simulink model "PID_Board"  (R2020b)
settings: Solver=ode3  StartTime=0.0  StopTime=inf  FixedStep=0.001  RelTol=1e-3  EnableMultiTasking=on
undefined symbols (not defined in the file or in its folder): Xgain, Xoffset
libraries: PoliArd x14, pid_lib x2, simulink x2
settings Model: ExtModeTrigDuration=2  Creator=User  LastModifiedBy=ernesto
settings DataIOCC: LimitDataPoints=on  SaveFormat=Array  ReturnWorkspaceOutputs=off
settings OptimizationCC: LifeSpan=1  EfficientTunableParamExpr=on
settings DebuggingCC: UnderspecifiedInitializationDetection=Classic  MergeDetectMultiDrivingBlocksExec=none  SFUnexpectedBacktrackingDiag=warning  SFNoUnconditionalDefaultTransitionDiag=warning  SFExecutionAtInitializationDiag=none  ArithmeticOperatorsInVariantConditions=warning
settings HardwareCC: ProdBitPerPointer=32  ProdBitPerSizeT=32  ProdBitPerPtrDiffT=32  ProdLargestAtomicInteger=Long  ProdLargestAtomicFloat=Double  ProdIntDivRoundTo=Undefined  ProdWordSize=32  ProdHWDeviceType=ARM Compatible->ARM Cortex
settings ModelReferenceCC: PropagateSignalLabelsOutOfModel=off
settings SFSimCC: SimUseLocalCustomCode=off  MATLABDynamicMemAlloc=off  CustomCodeUndefinedFunction=UseInterfaceOnly
settings RTWCC: Description=Run on Target Hardware  SystemTargetFile=realtime.tlc  GenerateMakefile=off  TemplateMakefile=realtime.tmf  RTWVerbose=off  RTWUseLocalCustomCode=off
settings CodeAppCC: StateflowObjectComments=on
settings STFCustomTargetCC: TargetLibSuffix=.a  GenerateSampleERTMain=on  ConcurrentExecutionCompliant=off  ERTCustomFileBanners=on  SupportNonInlinedSFcns=off  RemoveResetFunc=on  SupportVariableSizeSignals=on  MATLABClassNameForMDSCustomization=Simulink.SoftwareTarget.ERTCustomization  CPPClassGenCompliant=off  GRTInterface=off  SystemTargetFile=realtime.tlc
settings ERTTargetCC: MultiwordLength=2048  GenerateSampleERTMain=on  ParMdlRefBuildCompliant=off  CompOptLevelCompliant=off  ConcurrentExecutionCompliant=off  CombineOutputUpdateFcns=off  SupportContinuousTime=on  SupportVariableSizeSignals=on  ModelStepFunctionPrototypeControlCompliant=off  CPPClassGenCompliant=off  UseToolchainInfoCompliant=off  ExtModeTransport=3  ExtModeMexFile=ext_serial_win32_comm_rtt  ExtModeMexArgs=0 1 9600  ERTSrcFileBannerTemplate=realtime_code_template.cgt  ERTHdrFileBannerTemplate=realtime_code_template.cgt  ERTDataSrcFileTemplate=realtime_code_template.cgt  ERTDataHdrFileTemplate=realtime_code_template.cgt  ERTCustomFileTemplate=realtime_file_process.tlc  ConvertIfToSwitch=off  SuppressUnreachableDefaultCases=off
settings ConfigComp: CovMetricSettings=dw  CovSaveCumulativeToWorkspaceVar=on  CovSaveSingleToWorkspaceVar=on  CovExternalEMLEnable=off

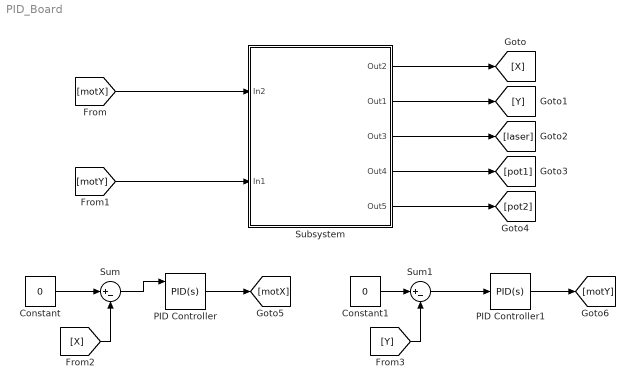
== system PID_Board ==
  Constant : Constant  Value=0
  Constant1 : Constant  Value=0
  PID Controller : pid_lib/PID Controller  Controller=PID  Form=Parallel  TimeDomain=Continuous-time  UseExternalTs=off  SampleTime=-1  IntegratorMethod=Forward Euler  FilterMethod=Forward Euler  ControllerParametersSource=external  P=1  I=1  D=0  UseFilter=on  N=100  TunerSelectOption=Transfer Function Based (PID Tuner App)  InitialConditionSource=internal  InitialConditionForIntegrator=0  InitialConditionForFilter=0  DifferentiatorICPrevScaledInput=0  ExternalReset=none  TrackingMode=off  Kt=1  LimitOutput=off  SatLimitsSource=internal  UpperSaturationLimit=inf  LowerSaturationLimit=-inf  LinearizeAsGain=on  AntiWindupMode=none  Kb=1  POutMin=[]  POutMax=[]  IOutMin=[]  IOutMax=[]  DOutMin=[]  DOutMax=[]  NOutMin=[]  NOutMax=[]  SumOutMin=[]  SumOutMax=[]  SaturationOutMin=[]  SaturationOutMax=[]  PParamMin=[]  PParamMax=[]  IParamMin=[]  IParamMax=[]  DParamMin=[]  DParamMax=[]  NParamMin=[]  NParamMax=[]  KbParamMin=[]  KbParamMax=[]  KtParamMin=[]  KtParamMax=[]  KbOutMin=[]  KbOutMax=[]  KtOutMin=[]  KtOutMax=[]  IntegratorOutMin=[]  IntegratorOutMax=[]  FilterOutMin=[]  FilterOutMax=[]  SumI1OutMin=[]  SumI1OutMax=[]  SumI2OutMin=[]  SumI2OutMax=[]  SumI3OutMin=[]  SumI3OutMax=[]  SumI4OutMin=[]  SumI4OutMax=[]  SumDOutMin=[]  SumDOutMax=[]  DifferentiatorOutMin=[]  DifferentiatorOutMax=[]  FilterDiffOutCoefMin=[]  FilterDiffOutCoefMax=[]  ReciprocalOutMin=[]  ReciprocalOutMax=[]  SumDenOutMin=[]  SumDenOutMax=[]  SumNumOutMin=[]  SumNumOutMax=[]  DivideOutMin=[]  DivideOutMax=[]  UdiffTsProdOutMin=[]  UdiffTsProdOutMax=[]  NTsProdOutMin=[]  NTsProdOutMax=[]  UintegralTsProdOutMin=[]  UintegralTsProdOutMax=[]  UngainTsProdOutMin=[]  UngainTsProdOutMax=[]  IntegratorContinuousStateAttributes=''  IntegratorStateMustResolveToSignalObject=off  IntegratorRTWStateStorageClass=Auto  FilterContinuousStateAttributes=''  FilterStateMustResolveToSignalObject=off  FilterRTWStateStorageClass=Auto  ParallelPVariant=ExternalParameters  IdealPVariant=Disabled  IVariant=ExternalParameters  DVariant=ExternalParameters  IntegratorVariant=Continuous  SatVariant=Disabled  AWVariant=Passthrough  PCopyVariant=Disabled  TRVariant=Disabled  FdbkBlocksVariant=Forward  IdealPFdbkVariant=Disabled  SatFdbkVariant=Disabled  DerivativeFilterVariant=ContFilter  NVariant=ExternalParameters  NCopyVariant=Disabled  FilterICVariant=InternalICsFilter  IntegratorICVariant=InternalICs  ExternalResetVariant=Disabled  TRSumVariant=Passthrough  SumFdbkVariant=Disabled  SumVariant=Sum_PID  TsampFilterVariant=InternalTs  TsampNgainVariant=Passthrough  TsampIntegralVariant=Passthrough  ExternalSaturationOutDataTypeStr=Inherit: Same as second input
  PID Controller1 : pid_lib/PID Controller  Controller=PID  Form=Parallel  TimeDomain=Continuous-time  UseExternalTs=off  SampleTime=-1  IntegratorMethod=Forward Euler  FilterMethod=Forward Euler  ControllerParametersSource=internal  P=1  I=1  D=0  UseFilter=on  N=100  TunerSelectOption=Transfer Function Based (PID Tuner App)  InitialConditionSource=internal  InitialConditionForIntegrator=0  InitialConditionForFilter=0  DifferentiatorICPrevScaledInput=0  ExternalReset=none  TrackingMode=off  Kt=1  LimitOutput=off  SatLimitsSource=internal  UpperSaturationLimit=inf  LowerSaturationLimit=-inf  LinearizeAsGain=on  AntiWindupMode=none  Kb=1  POutMin=[]  POutMax=[]  IOutMin=[]  IOutMax=[]  DOutMin=[]  DOutMax=[]  NOutMin=[]  NOutMax=[]  SumOutMin=[]  SumOutMax=[]  SaturationOutMin=[]  SaturationOutMax=[]  PParamMin=[]  PParamMax=[]  IParamMin=[]  IParamMax=[]  DParamMin=[]  DParamMax=[]  NParamMin=[]  NParamMax=[]  KbParamMin=[]  KbParamMax=[]  KtParamMin=[]  KtParamMax=[]  KbOutMin=[]  KbOutMax=[]  KtOutMin=[]  KtOutMax=[]  IntegratorOutMin=[]  IntegratorOutMax=[]  FilterOutMin=[]  FilterOutMax=[]  SumI1OutMin=[]  SumI1OutMax=[]  SumI2OutMin=[]  SumI2OutMax=[]  SumI3OutMin=[]  SumI3OutMax=[]  SumI4OutMin=[]  SumI4OutMax=[]  SumDOutMin=[]  SumDOutMax=[]  DifferentiatorOutMin=[]  DifferentiatorOutMax=[]  FilterDiffOutCoefMin=[]  FilterDiffOutCoefMax=[]  ReciprocalOutMin=[]  ReciprocalOutMax=[]  SumDenOutMin=[]  SumDenOutMax=[]  SumNumOutMin=[]  SumNumOutMax=[]  DivideOutMin=[]  DivideOutMax=[]  UdiffTsProdOutMin=[]  UdiffTsProdOutMax=[]  NTsProdOutMin=[]  NTsProdOutMax=[]  UintegralTsProdOutMin=[]  UintegralTsProdOutMax=[]  UngainTsProdOutMin=[]  UngainTsProdOutMax=[]  IntegratorContinuousStateAttributes=''  IntegratorStateMustResolveToSignalObject=off  IntegratorRTWStateStorageClass=Auto  FilterContinuousStateAttributes=''  FilterStateMustResolveToSignalObject=off  FilterRTWStateStorageClass=Auto  ParallelPVariant=InternalParameters  IdealPVariant=Disabled  IVariant=InternalParameters  DVariant=InternalParameters  IntegratorVariant=Continuous  SatVariant=Disabled  AWVariant=Passthrough  PCopyVariant=Disabled  TRVariant=Disabled  FdbkBlocksVariant=Forward  IdealPFdbkVariant=Disabled  SatFdbkVariant=Disabled  DerivativeFilterVariant=ContFilter  NVariant=InternalParameters  NCopyVariant=Disabled  FilterICVariant=InternalICsFilter  IntegratorICVariant=InternalICs  ExternalResetVariant=Disabled  TRSumVariant=Passthrough  SumFdbkVariant=Disabled  SumVariant=Sum_PID  TsampFilterVariant=InternalTs  TsampNgainVariant=Passthrough  TsampIntegralVariant=Passthrough  ExternalSaturationOutDataTypeStr=Inherit: Same as second input
  Subsystem : Subsystem
  Sum : Sum  Inputs=|+-
  Sum1 : Sum  Inputs=|+-
  wires:
  [motX] -> Subsystem/1(In2)
  [motY] -> Subsystem/2(In1)
  Subsystem/2(Out1) -> [Y]
  Subsystem/1(Out2) -> [X]
  Subsystem/3(Out3) -> [laser]
  Subsystem/4(Out4) -> [pot1]
  Subsystem/5(Out5) -> [pot2]
  [X] -> Sum/2
  Sum/1 -> PID Controller/1
  PID Controller/1 -> [motX]
  Constant/1 -> Sum/1
  PID Controller1/1 -> [motY]
  Sum1/1 -> PID Controller1/1
  Constant1/1 -> Sum1/1
  [Y] -> Sum1/2

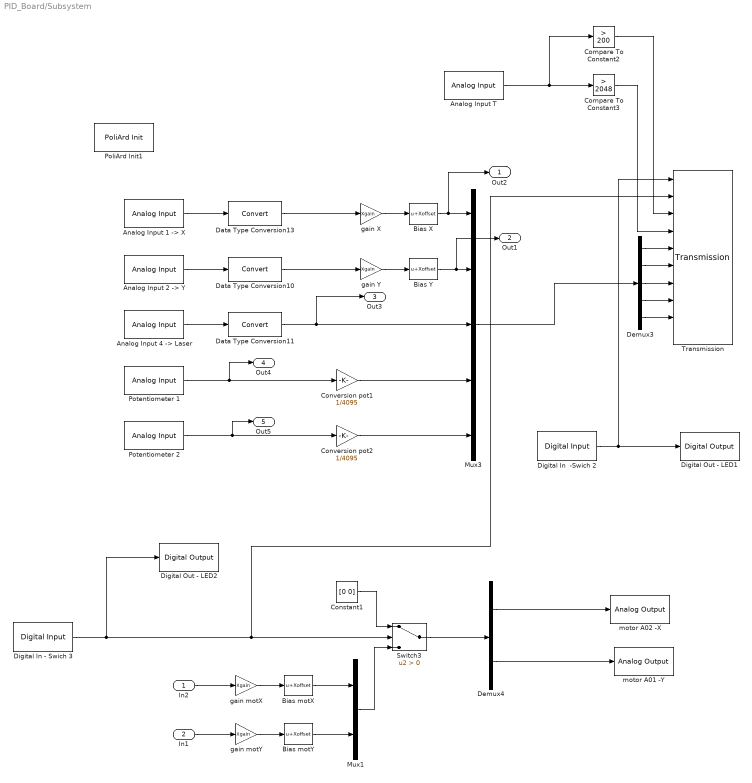
== system PID_Board/Subsystem ==
  In2 : Inport
  In1 : Inport  Port=2
  "Analog Input 1 -> X" : PoliArd/Analog Input  AIpin_mask=1  AIsample=-1
  "Analog Input 2 -> Y" : PoliArd/Analog Input  AIpin_mask=2  AIsample=-1
  "Analog Input 4 -> Laser" : PoliArd/Analog Input  AIpin_mask=4  AIsample=-1
  Analog Input T : PoliArd/Analog Input  AIpin_mask=7  AIsample=-1
  Bias X : Bias  Bias=Xoffset
  Bias Y : Bias  Bias=Xoffset
  Bias motX : Bias  Bias=Xoffset
  Bias motY : Bias  Bias=Xoffset
  Compare To Constant2 : simulink/Logic and Bit Operations/Compare To Constant  relop=>  const=200  OutDataTypeStr=boolean
  Compare To Constant3 : simulink/Logic and Bit Operations/Compare To Constant  relop=>  const=2048  OutDataTypeStr=boolean
  Constant1 : Constant  Value=[0 0]
  Conversion pot1 : Gain  Gain=1/4095
  Conversion pot2 : Gain  Gain=1/4095
  Data Type Conversion10 : DataTypeConversion
  Data Type Conversion11 : DataTypeConversion
  Data Type Conversion13 : DataTypeConversion
  Demux3 : Demux  Outputs=5
  Demux4 : Demux  Outputs=2
  Digital In  -Swich 2 : PoliArd/Digital Input  DI_pin=2  DIsample=-1
  Digital In - Swich 3 : PoliArd/Digital Input  DI_pin=3  DIsample=-1
  Digital Out - LED1 : PoliArd/Digital Output  DO_pin=1
  Digital Out - LED2 : PoliArd/Digital Output  DO_pin=2
  Mux1 : Mux  Inputs=2
  Mux3 : Mux  Inputs=5
  PoliArd Init1 : PoliArd/PoliArd Init
  Potentiometer 1 : PoliArd/Analog Input  AIpin_mask=8  AIsample=-1
  Potentiometer 2 : PoliArd/Analog Input  AIpin_mask=9  AIsample=-1
  Switch3 : Switch  Criteria=u2 > Threshold
  Transmission : PoliArd/Transmission  sample_freq=100  sig_to_send=6
  gain X : Gain  Gain=Xgain
  gain Y : Gain  Gain=Xgain
  gain motX : Gain  Gain=Xgain
  gain motY : Gain  Gain=Xgain
  motor A01 -Y : PoliArd/Analog Output  DAC_pin_mask=2
  motor A02 -X : PoliArd/Analog Output  DAC_pin_mask=1
  Out2 : Outport
  Out1 : Outport  Port=2
  Out3 : Outport  Port=3
  Out4 : Outport  Port=4
  Out5 : Outport  Port=5
  wires:
  Potentiometer 1/1 -> Conversion pot1/1, Out4/1
  Digital In - Swich 3/1 -> Digital Out - LED2/1, Transmission/2, Switch3/2
  "Analog Input 1 -> X"/1 -> Data Type Conversion13/1
  Mux1/1 -> Switch3/3
  Switch3/1 -> Demux4/1
  Mux3/1 -> Demux3/1
  Compare To Constant3/1 -> Transmission/4
  Demux3/3 -> Transmission/7
  Constant1/1 -> Switch3/1
  Demux3/1 -> Transmission/5
  Demux4/2 -> motor A01 -Y/1
  Demux3/4 -> Transmission/8
  Demux4/1 -> motor A02 -X/1
  Potentiometer 2/1 -> Conversion pot2/1, Out5/1
  Analog Input T/1 -> Compare To Constant3/1, Compare To Constant2/1
  Demux3/5 -> Transmission/9
  Data Type Conversion11/1 -> Out3/1, Mux3/3
  Digital In  -Swich 2/1 -> Digital Out - LED1/1, Transmission/1
  Data Type Conversion10/1 -> gain Y/1
  "Analog Input 2 -> Y"/1 -> Data Type Conversion10/1
  Demux3/2 -> Transmission/6
  Compare To Constant2/1 -> Transmission/3
  Data Type Conversion13/1 -> gain X/1
  "Analog Input 4 -> Laser"/1 -> Data Type Conversion11/1
  Conversion pot2/1 -> Mux3/5
  Conversion pot1/1 -> Mux3/4
  gain X/1 -> Bias X/1
  Bias X/1 -> Out2/1, Mux3/1
  gain Y/1 -> Bias Y/1
  Bias Y/1 -> Out1/1, Mux3/2
  In2/1 -> gain motX/1
  In1/1 -> gain motY/1
  Bias motX/1 -> Mux1/1
  gain motX/1 -> Bias motX/1
  Bias motY/1 -> Mux1/2
  gain motY/1 -> Bias motY/1
